simulink model "BPSKDemo"  (R2018b)
settings: Solver=VariableStepAuto  StartTime=0.0  StopTime=10.0  RelTol=1e-3
libraries: peGeneralControl x2, simulink x1
settings Model: Creator=hp  LastModifiedBy=hp

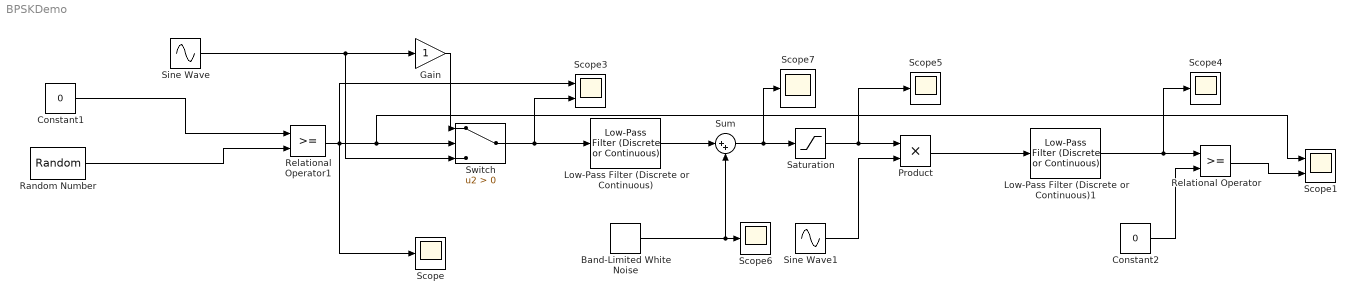
== system BPSKDemo ==
  Band-Limited White Noise : simulink/Sources/Band-Limited White Noise  Cov=[0.1]  Ts=0.1  seed=[23341]
  Constant1 : Constant  Value=0
  Constant2 : Constant  Value=0
  Gain : Gain
  Low-Pass Filter (Discrete or Continuous) : peGeneralControl/Low-Pass Filter (Discrete or Continuous)  K=1  T=1  B=inf  A=-inf  Ts=-1
  Low-Pass Filter (Discrete or Continuous)1 : peGeneralControl/Low-Pass Filter (Discrete or Continuous)  K=1  T=1  B=inf  A=-inf  Ts=-1
  Product : Product
  Random Number : RandomNumber  SampleTime=0.1
  Relational Operator : RelationalOperator  OutDataTypeStr=boolean  RndMeth=Simplest
  Relational Operator1 : RelationalOperator  OutDataTypeStr=boolean  RndMeth=Simplest
  Saturation : Saturate
  Scope{,4..7} (5 alike) : Scope
  Scope1 : Scope  NumInputPorts=2
  Scope3 : Scope  NumInputPorts=2
  Sine Wave : Sin  SampleTime=0
  Sine Wave1 : Sin  SampleTime=0
  Sum : Sum  Inputs=|++
  Switch : Switch  Criteria=u2 > Threshold
  wires:
  Random Number/1 -> Relational Operator1/2
  Constant1/1 -> Relational Operator1/1
  Sine Wave/1 -> Switch/3, Gain/1
  Relational Operator1/1 -> Scope3/1, Scope/1, Switch/2, Scope1/1
  Gain/1 -> Switch/1
  Switch/1 -> Low-Pass Filter (Discrete or Continuous)/1, Scope3/2
  Saturation/1 -> Scope5/1, Product/1
  Sine Wave1/1 -> Product/2
  Product/1 -> Low-Pass Filter (Discrete or Continuous)1/1
  Low-Pass Filter (Discrete or Continuous)1/1 -> Scope4/1, Relational Operator/1
  Constant2/1 -> Relational Operator/2
  Relational Operator/1 -> Scope1/2
  Low-Pass Filter (Discrete or Continuous)/1 -> Sum/1
  Band-Limited White Noise/1 -> Scope6/1, Sum/2
  Sum/1 -> Scope7/1, Saturation/1
